simulink model "aircraft_lqr"  (R2018b)
settings: Solver=VariableStepAuto  StartTime=0.0  StopTime=10  RelTol=1e-3
settings Model: Creator=adelina  LastModifiedBy=adelina

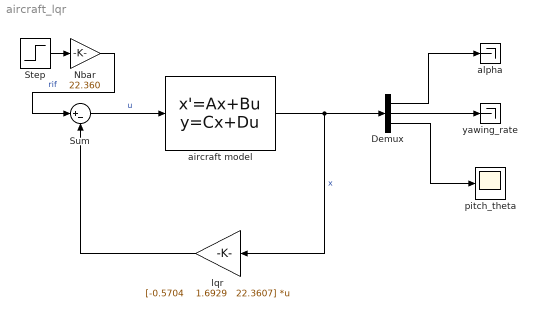
== system aircraft_lqr ==
  Demux : Demux  Outputs=3
  Nbar : Gain  Gain=22.360
  Step : Step  After=0.5  SampleTime=0
  Sum : Sum  Inputs=|+-
  aircraft model : StateSpace  A=[-2.02 1 0; -6.9868 -2.9476 0; 0 1 0]  B=[0.16; 11.7304; 0]  C=eye(3)  D=[0;0;0]  InitialCondition=0  ContinuousStateAttributes={'alpha', 'yawing_rate', 'pitch_theta'}
  alpha : Terminator
  lqr : Gain  Gain="[-0.5704    1.6929   22.3607]"  Multiplication=Matrix(K*u)
  pitch_theta : Scope
  yawing_rate : Terminator
  wires:
  lqr/1 -> Sum/2
  Sum/1 -> aircraft model/1  "u"
  aircraft model/1 -> lqr/1, Demux/1  "x"
  Demux/3 -> pitch_theta/1
  Demux/1 -> alpha/1
  Demux/2 -> yawing_rate/1
  Step/1 -> Nbar/1
  Nbar/1 -> Sum/1  "rif"
